simulink model "Front_control"  (R2025b)
settings: Solver=VariableStepAuto  StartTime=0.0  StopTime=60  RelTol=1e-3
undefined symbols (not defined in the file): A, B, C, k, Nu, Nx
settings Model: Creator=lilkiddy  LastModifiedBy=lilkiddy

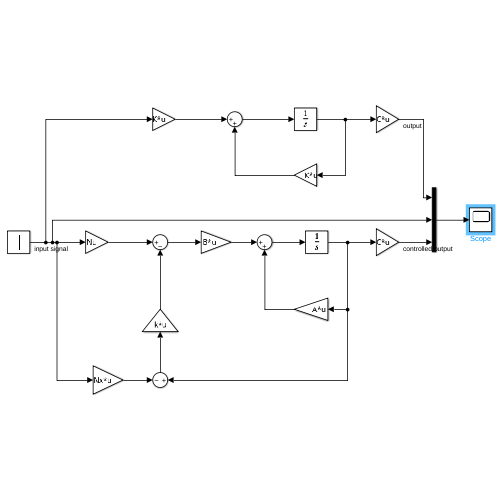
[thumbnail: Simulink's stored preview of the top-level diagram]
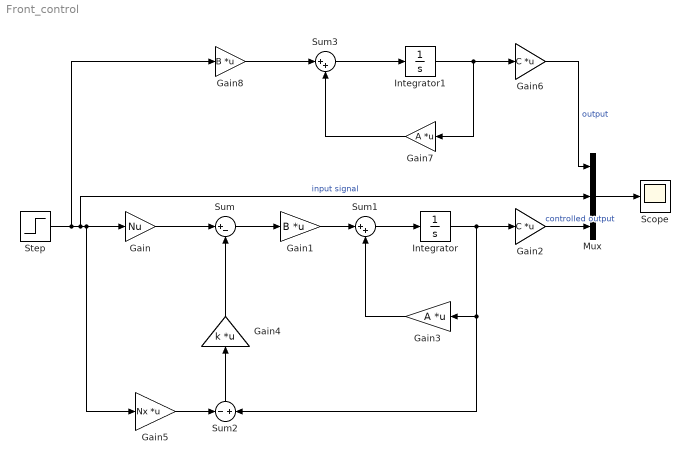
== system Front_control ==
  Gain : Gain  Gain=Nu
  Gain1 : Gain  Gain=B  Multiplication=Matrix(K*u)
  Gain2 : Gain  Gain=C  Multiplication=Matrix(K*u)
  Gain3 : Gain  Gain=A  Multiplication=Matrix(K*u)
  Gain4 : Gain  Gain=k  Multiplication=Matrix(K*u)
  Gain5 : Gain  Gain=Nx  Multiplication=Matrix(K*u)
  Gain6 : Gain  Gain=C  Multiplication=Matrix(K*u)
  Gain7 : Gain  Gain=A  Multiplication=Matrix(K*u)
  Gain8 : Gain  Gain=B  Multiplication=Matrix(K*u)
  Integrator : Integrator
  Integrator1 : Integrator
  Mux : Mux  Inputs=3
  Scope : Scope
      settings: ActiveDisplayYMinimum=-0.17959161080321717  ActiveDisplayYMaximum=1.6163244972289548  YLabel=displacement
  Step : Step  SampleTime=0
  Sum : Sum  Inputs=|+-
  Sum1 : Sum  Inputs=|++
  Sum2 : Sum  Inputs=-|+
  Sum3 : Sum  Inputs=|++
  wires:
  Step/1 -> Gain8/1, Mux/2, Gain5/1, Gain/1  "input signal"
  Gain/1 -> Sum/1
  Sum/1 -> Gain1/1
  Gain1/1 -> Sum1/1
  Sum1/1 -> Integrator/1
  Integrator/1 -> Sum2/2, Gain3/1, Gain2/1
  Gain3/1 -> Sum1/2
  Gain4/1 -> Sum/2
  Mux/1 -> Scope/1
  Gain2/1 -> Mux/3  "controlled output"
  Sum2/1 -> Gain4/1
  Gain5/1 -> Sum2/1
  Gain6/1 -> Mux/1  "output"
  Integrator1/1 -> Gain7/1, Gain6/1
  Sum3/1 -> Integrator1/1
  Gain7/1 -> Sum3/2
  Gain8/1 -> Sum3/1
